simulink model "odev2 (2)"  (R2013a)
settings: Solver=ode45  StartTime=0.0  StopTime=10.0  RelTol=1e-3
undefined symbols (not defined in the file): jet, Rec, SDTV
libraries: visionconversions x4, visionsources x1, visionsinks x1
settings Model: Creator=bizimakin  LastModifiedBy=bizimakin

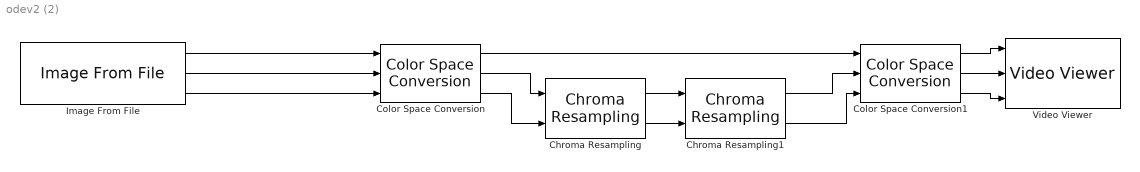
== system odev2 (2) ==
  Chroma Resampling : visionconversions/Chroma Resampling  resampling=4:4:4 to 4:2:2  interpolation=pixel replication  antialiasing=Default  hcoeff=[0.2 0.6 0.2]  vcoeff=[0.5 0.5]  isInputTransposed=off
  Chroma Resampling1 : visionconversions/Chroma Resampling  resampling=4:2:2 to 4:4:4  interpolation=linear  antialiasing=Default  hcoeff=[0.2 0.6 0.2]  vcoeff=[0.5 0.5]  isInputTransposed=off
  Color Space Conversion : visionconversions/Color Space  Conversion  conversion=Obsolete  conversionActive=R'G'B' to Y'CbCr  wp_str=D65  rec=Rec. 601 (SDTV)  sys=1125/60/2:1  imagePorts=Separate color signals
  Color Space Conversion1 : visionconversions/Color Space  Conversion  conversion=Obsolete  conversionActive=Y'CbCr to R'G'B'  wp_str=D65  rec=Rec. 601 (SDTV)  sys=1125/60/2:1  imagePorts=Separate color signals
  Image From File : visionsources/Image From File  Tag=vipblks_nd  FileName=peppers.png  imagePorts=Separate color signals  Ts=inf  ImageDataType=double  Signed=on  WordLength=16  sdImageDataType=uint(8)  FractionLengthMode=User-defined  FractionLength=15  OutPortLabels=R|G|B
  Video Viewer : visionsinks/Video Viewer  inputType=Obsolete7b  imagePorts=Separate color signals  useColorMap=off  colormapValue=jet(256)  specRange=off  minInputVal=0  maxInputVal=255  FigPos=[163 697 410 300]  AxisZoom=on  trueSizedOnce=off  OpenAtMdlStart=on  DefaultConfigurationName=vipscopes.VideoViewerScopeCfg
  wires:
  Color Space Conversion/1 -> Color Space Conversion1/1
  Color Space Conversion/2 -> Chroma Resampling/1
  Color Space Conversion/3 -> Chroma Resampling/2
  Color Space Conversion1/1 -> Video Viewer/1
  Chroma Resampling/1 -> Chroma Resampling1/1
  Chroma Resampling/2 -> Chroma Resampling1/2
  Color Space Conversion1/2 -> Video Viewer/2
  Color Space Conversion1/3 -> Video Viewer/3
  Chroma Resampling1/1 -> Color Space Conversion1/2
  Chroma Resampling1/2 -> Color Space Conversion1/3
  Image From File/2 -> Color Space Conversion/2
  Image From File/3 -> Color Space Conversion/3
  Image From File/1 -> Color Space Conversion/1
